simulink model "vexv5_Record_Motion"  (R2019b)
settings: Solver=ode3  StartTime=0.0  StopTime=inf  RelTol=1e-3  EnableMultiTasking=on
libraries: vexv5lib x9, vexcommonlib x1, vexv5_SD_Logging_Lib x1
settings Model: SimulationMode=external  ExtModeTrigDuration=5  Creator=The MathWorks, Inc.  LastModifiedBy=josea
settings DataIOCC: LimitDataPoints=on  SaveFormat=Array  ReturnWorkspaceOutputs=off
settings OptimizationCC: ExpressionDepthLimit=2147483647  LifeSpan=Inf  MaxStackSize=64  EfficientTunableParamExpr=on
settings DebuggingCC: UnderspecifiedInitializationDetection=Classic  MergeDetectMultiDrivingBlocksExec=none  InheritedTsInSrcMsg=none  FcnCallInpInsideContextMsg=warning  UnconnectedInputMsg=none  UnconnectedOutputMsg=none  AllowSymbolicDim=off  StateNameClashWarn=warning  SFUnexpectedBacktrackingDiag=warning  SFNoUnconditionalDefaultTransitionDiag=warning  SFExecutionAtInitializationDiag=none  ArithmeticOperatorsInVariantConditions=warning
settings HardwareCC: ProdBitPerPointer=32  ProdBitPerSizeT=32  ProdBitPerPtrDiffT=32  ProdLargestAtomicInteger=Long  ProdLargestAtomicFloat=Double  ProdWordSize=32  ProdHWDeviceType=ARM Compatible->ARM Cortex
settings ModelReferenceCC: PropagateSignalLabelsOutOfModel=off
settings SFSimCC: SimUseLocalCustomCode=off  CustomCodeUndefinedFunction=UseInterfaceOnly
settings RTWCC: SystemTargetFile=ert.tlc  HardwareBoard=VEX V5 Robot Brain  TLCOptions=-aInlineSetEventsForThisBaseRateFcn=TLC_FALSE -aSuppressMultiTaskScheduler=TLC_FALSE -aRateBasedStepFcn=0  TemplateMakefile=ert_default_tmf  RTWUseLocalCustomCode=off  Toolchain=GNU Tools for ARM Embedded Processors
settings CodeAppCC: StateflowObjectComments=on
settings ERTTargetCC: CodeReplacementLibrary=GCC ARM Cortex-M3  MultiwordLength=2048  ERTCustomFileBanners=off  MatFileLogging=on  SupportContinuousTime=on  SupportNonInlinedSFcns=on  RemoveResetFunc=off  ModelStepFunctionPrototypeControlCompliant=off  ConvertIfToSwitch=off  SuppressUnreachableDefaultCases=off
settings ConfigComp: CovMetricSettings=dw  CovHtmlReporting=on  CovSaveCumulativeToWorkspaceVar=on  CovSaveSingleToWorkspaceVar=on  CovExternalEMLEnable=off  CovSFcnEnable=off

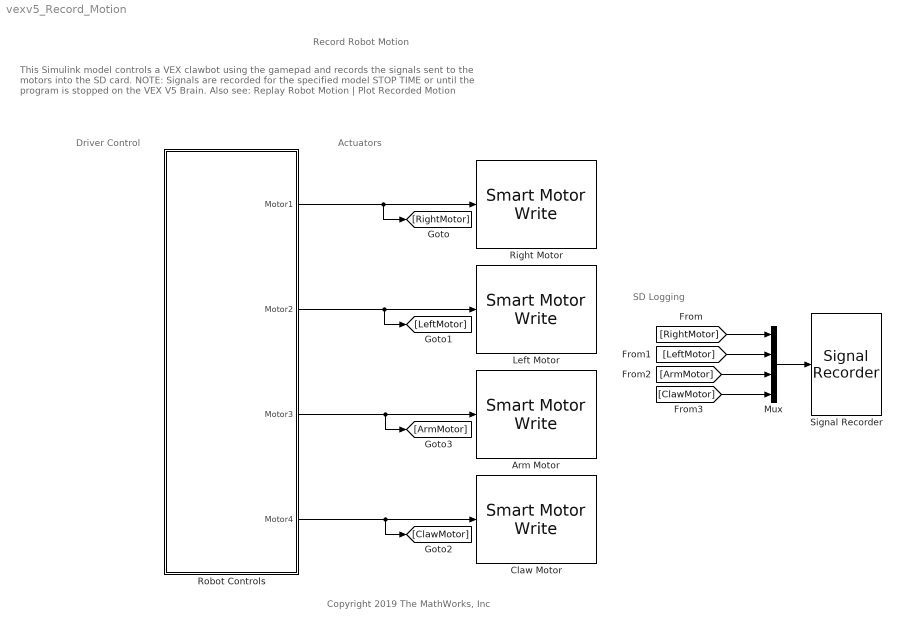
== system vexv5_Record_Motion ==
  note: Driver Control
  note: SD Logging
  note: Actuators
  note: Copyright 2019 The MathWorks, Inc
  note: Record Robot Motion
  note: This Simulink model controls a VEX clawbot using the gamepad and records the signals sent to the motors into the SD card.
      | NOTE: Signals are recorded for the specified model STOP TIME or until the program is stopped on the VEX V5 Brain.
      |
      | Also see: Replay Robot Motion | Plot Recorded Motion
  Arm Motor : vexv5lib/Actuators/Smart Motor Write  motorPort=8  scaleFactor=18:1  MotorBrakeMode=Hold  OperationMode=Velocity Control
      settings: SourceProductName=Simulink Coder Support Package for VEX EDR V5 Robot Brain
  Claw Motor : vexv5lib/Actuators/Smart Motor Write  motorPort=3  scaleFactor=18:1  MotorBrakeMode=Hold  OperationMode=Velocity Control
      settings: SourceProductName=Simulink Coder Support Package for VEX EDR V5 Robot Brain
  Left Motor : vexv5lib/Actuators/Smart Motor Write  motorPort=1  scaleFactor=18:1  MotorBrakeMode=Coast  OperationMode=Velocity Control
      settings: SourceProductName=Simulink Coder Support Package for VEX EDR V5 Robot Brain
  Mux : Mux
  Right Motor : vexv5lib/Actuators/Smart Motor Write  motorPort=10  scaleFactor=18:1  MotorBrakeMode=Coast  OperationMode=Velocity Control
      settings: SourceProductName=Simulink Coder Support Package for VEX EDR V5 Robot Brain
  Robot Controls : Subsystem
  Signal Recorder : vexv5_SD_Logging_Lib/Signal Recorder  SampleTime=-1
  wires:
  [RightMotor] -> Mux/1
  [LeftMotor] -> Mux/2
  [ArmMotor] -> Mux/3
  [ClawMotor] -> Mux/4
  Mux/1 -> Signal Recorder/1
  Robot Controls/1(Motor1) -> [RightMotor], Right Motor/1
  Robot Controls/4(Motor4) -> [ClawMotor], Claw Motor/1
  Robot Controls/2(Motor2) -> [LeftMotor], Left Motor/1
  Robot Controls/3(Motor3) -> [ArmMotor], Arm Motor/1

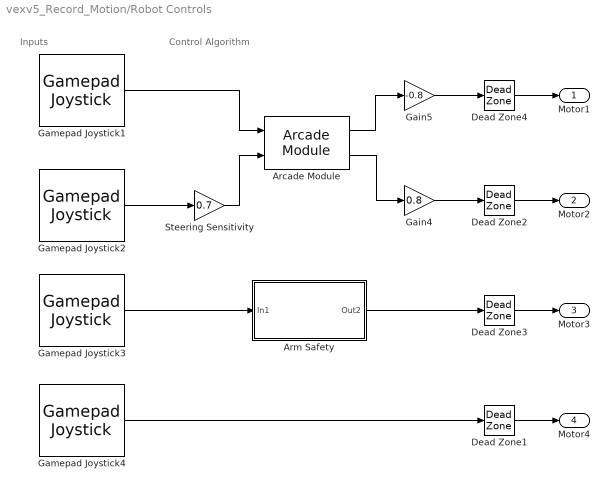
== system vexv5_Record_Motion/Robot Controls ==
  note: Control Algorithm
  note: Inputs
  Arcade Module : vexcommonlib/Arcade Module  BlockPlatform=vexarmcortex
      settings: SourceProductName=Simulink Coder Support Package for ARM Cortex-based VEX Microcontroller  SourceProductBaseCode=EC_VEX_MICRO
  Arm Safety : Subsystem
  Dead Zone{1..4} (4 alike) : DeadZone  LowerValue=-5  UpperValue=5  SaturateOnIntegerOverflow=on
  Gain4 : Gain  Gain=0.8
  Gain5 : Gain  Gain=-0.8
  Gamepad Joystick1 : vexv5lib/Gamepad/Gamepad Joystick  joystickType=Master  chan=3  SampleTime=0.02
      settings: SourceProductName=Simulink Coder Support Package for VEX EDR V5 Robot Brain
  Gamepad Joystick2 : vexv5lib/Gamepad/Gamepad Joystick  joystickType=Master  chan=4  SampleTime=0.02
      settings: SourceProductName=Simulink Coder Support Package for VEX EDR V5 Robot Brain
  Gamepad Joystick3 : vexv5lib/Gamepad/Gamepad Joystick  joystickType=Master  chan=2  SampleTime=0.02
      settings: SourceProductName=Simulink Coder Support Package for VEX EDR V5 Robot Brain
  Gamepad Joystick4 : vexv5lib/Gamepad/Gamepad Joystick  joystickType=Master  chan=1  SampleTime=0.02
      settings: SourceProductName=Simulink Coder Support Package for VEX EDR V5 Robot Brain
  Steering Sensitivity : Gain  Gain=0.7
  Motor1 : Outport
  Motor2 : Outport  Port=2
  Motor3 : Outport  Port=3
  Motor4 : Outport  Port=4
  wires:
  Arm Safety/1(Out2) -> Dead Zone3/1
  Gamepad Joystick2/1 -> Steering Sensitivity/1
  Gamepad Joystick3/1 -> Arm Safety/1(In1)
  Gain4/1 -> Dead Zone2/1
  Arcade Module/1 -> Gain5/1
  Gamepad Joystick4/1 -> Dead Zone1/1
  Gamepad Joystick1/1 -> Arcade Module/1
  Gain5/1 -> Dead Zone4/1
  Steering Sensitivity/1 -> Arcade Module/2
  Arcade Module/2 -> Gain4/1
  Dead Zone1/1 -> Motor4/1
  Dead Zone2/1 -> Motor2/1
  Dead Zone4/1 -> Motor1/1
  Dead Zone3/1 -> Motor3/1

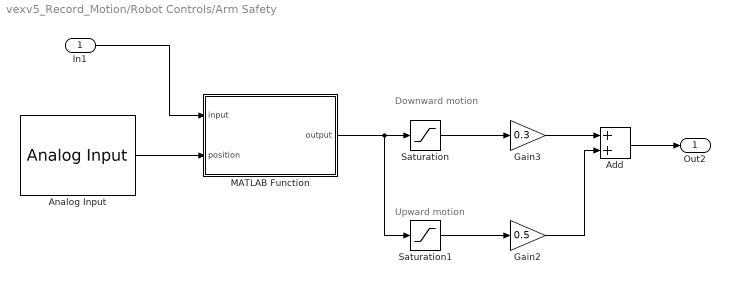
== system vexv5_Record_Motion/Robot Controls/Arm Safety ==
  note: Downward motion
  note: Upward motion
  In1 : Inport
  Add : Sum
  Analog Input : vexv5lib/Sensors/Analog Input  port=A  SampleTime=0.02
      settings: SourceProductName=Simulink Coder Support Package for VEX EDR V5 Robot Brain
  Gain2 : Gain  Gain=0.5
  Gain3 : Gain  Gain=0.3
  MATLAB Function : MATLAB Function  TreatAsAtomicUnit=on
  Saturation : Saturate  UpperLimit=0  LowerLimit=-127
  Saturation1 : Saturate  UpperLimit=127  LowerLimit=0
  Out2 : Outport  VectorParamsAs1DForOutWhenUnconnected=off
  wires:
  Gain2/1 -> Add/2
  Add/1 -> Out2/1
  Saturation/1 -> Gain3/1
  Saturation1/1 -> Gain2/1
  Gain3/1 -> Add/1
  MATLAB Function/1(output) -> Saturation1/1, Saturation/1
  In1/1 -> MATLAB Function/1(input)
  Analog Input/1 -> MATLAB Function/2(position)

== matlab function vexv5_Record_Motion/Robot Controls/Arm Safety/MATLAB Function ==
  data: input input; output output; position input
function output = armLimits(input, position)

if input >0 && position < 2650
    output=input;
elseif input <0 && position > 1400
    output=input;
else
    output=0;
end

end
